simulink model "hoist"  (R2023b)
settings: Solver=FixedStepAuto  StartTime=0.0  StopTime=10.0  FixedStep=0.001  RelTol=1e-3
undefined symbols (not defined in the file): b_hb, b_hEb, b_hwu, bh_eq, i_h, Jh_eq, K_hwu, L_h0, r_hd, T_hb_max, T_hEb_max, Y_t0
settings Model: Creator=Ferran  LastModifiedBy=Ferran
settings DebuggingCC: AlgebraicLoopMsg=none  ArtificialAlgebraicLoopMsg=none
settings ModelReferenceCC: ModelReferenceMinAlgLoopOccurrences=on

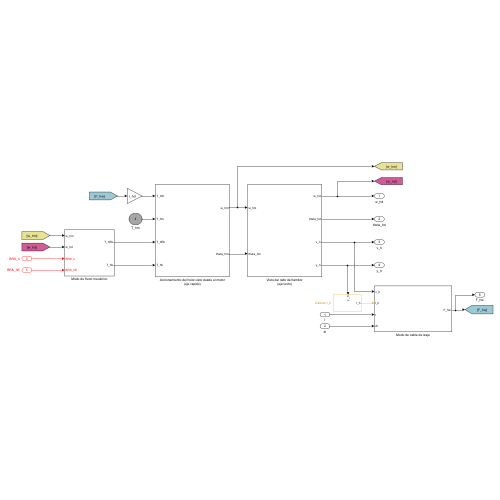
[thumbnail: Simulink's stored preview of the top-level diagram]
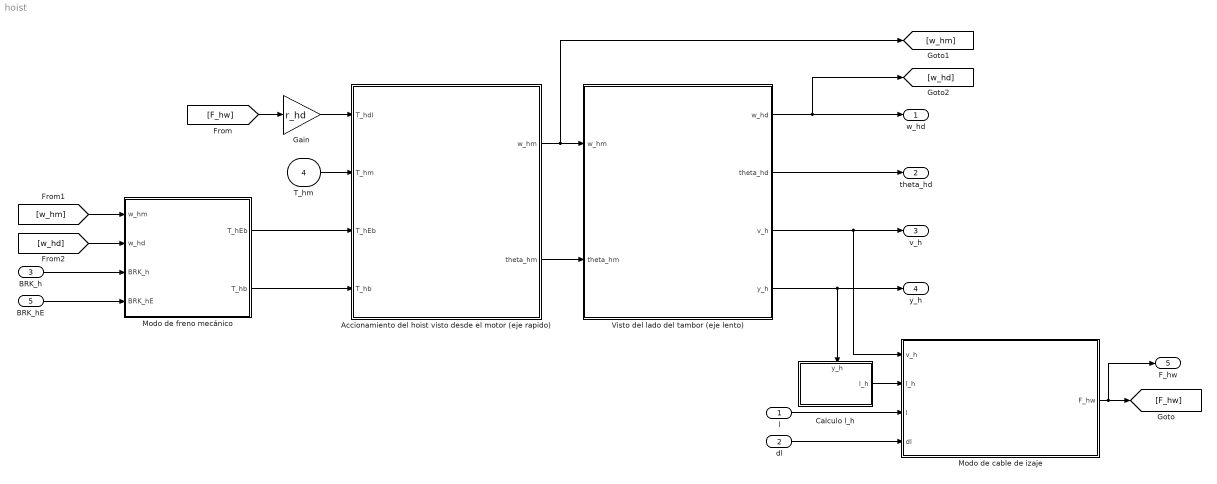
== system hoist ==
  l : Inport
  dl : Inport  Port=2
  BRK_h : Inport  Port=3
  T_hm : Inport  Port=4
  BRK_hE : Inport  Port=5
  Accionamiento del hoist visto desde el motor (eje rapido) : Subsystem
  Calculo l_h : Subsystem
      settings: PortSchema="{\"entries\":[{\"content\":{\"sides\":[{\"content\":{\"connectorIds\":[\"Out1\"]},\"type\":\"ConnectorPlacement.EquallySpacedRectSide\",\"uuid\":\"07ea2d8b-a4bd-4a00-9f3e-d3723522cead\"},{\"content\":{\"side\":\"RIGHT\"},\"type\":\"ConnectorPlacement.EquallySpacedRectSide\",\"uuid\":\"e7371649-c13b-4c3e-a52c-6db8f2f471a9\"},{\"content\":{\"side\":\"TOP\"},\"type\":\"ConnectorPlacement.EquallySpacedRectSide\",\"uuid\":\"bf44ddc9-8ab8-43a2-b974-62ce3b2d20dc\"},{\"content\":{\"connectorIds\":[\"In1\"],\"side\":\"BOTTOM\"},\"type\":\"ConnectorPlacement.EquallySpacedRectSide\",\"uuid\":\"68df679a-1ec0-4ce0-a9ee-39677e661654\"}]},\"type\":\"ConnectorPlacement.EquallySpacedConnector\",\"uuid\":\"345e5710-5df9-4bf4-96c9-62f27951d1e0\"}],\"packageUris\":[\"http://schema.mathworks.com/mf0/Connector/R2020b\"],\"version\":\"1.0\"}"
  Gain : Gain  Gain=r_hd
  Modo de cable de izaje : Subsystem
  Modo de freno mecánico : Subsystem
  Visto del lado del tambor (eje lento) : Subsystem
  w_hd : Outport
  theta_hd : Outport  Port=2
  v_h : Outport  Port=3
  y_h : Outport  Port=4
  F_hw : Outport  Port=5
  wires:
  Accionamiento del hoist visto desde el motor (eje rapido)/2(theta_hm) -> Visto del lado del tambor (eje lento)/2(theta_hm)
  Accionamiento del hoist visto desde el motor (eje rapido)/1(w_hm) -> Visto del lado del tambor (eje lento)/1(w_hm), [w_hm]
  Visto del lado del tambor (eje lento)/4(y_h) -> y_h/1, Calculo l_h/1(y_h)
  l/1 -> Modo de cable de izaje/3(l)
  Calculo l_h/1(l_h) -> Modo de cable de izaje/2(l_h)
  Visto del lado del tambor (eje lento)/3(v_h) -> v_h/1, Modo de cable de izaje/1(v_h)
  Modo de cable de izaje/1(F_hw) -> F_hw/1, [F_hw]
  [F_hw] -> Gain/1
  Gain/1 -> Accionamiento del hoist visto desde el motor (eje rapido)/1(T_hdl)
  dl/1 -> Modo de cable de izaje/4(dl)
  T_hm/1 -> Accionamiento del hoist visto desde el motor (eje rapido)/2(T_hm)
  Visto del lado del tambor (eje lento)/1(w_hd) -> [w_hd], w_hd/1
  Visto del lado del tambor (eje lento)/2(theta_hd) -> theta_hd/1
  BRK_hE/1 -> Modo de freno mecánico/4(BRK_hE)
  [w_hd] -> Modo de freno mecánico/2(w_hd)
  BRK_h/1 -> Modo de freno mecánico/3(BRK_h)
  [w_hm] -> Modo de freno mecánico/1(w_hm)
  Modo de freno mecánico/1(T_hEb) -> Accionamiento del hoist visto desde el motor (eje rapido)/3(T_hEb)
  Modo de freno mecánico/2(T_hb) -> Accionamiento del hoist visto desde el motor (eje rapido)/4(T_hb)

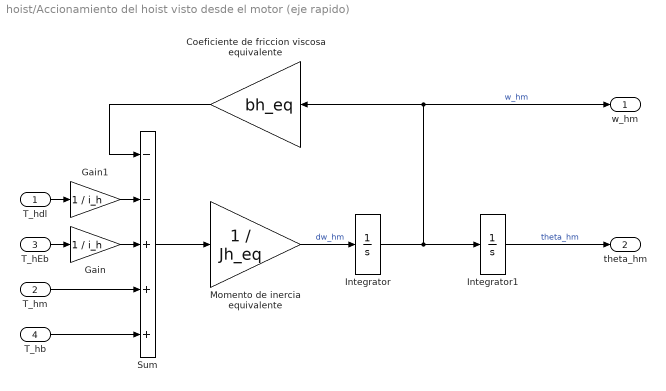
== system hoist/Accionamiento del hoist visto desde el motor (eje rapido) ==
  T_hdl : Inport
  T_hm : Inport  Port=2
  T_hEb : Inport  Port=3
  T_hb : Inport  Port=4
  Coeficiente de friccion viscosa equivalente : Gain  Gain=bh_eq
  Gain : Gain  Gain=1 / i_h
  Gain1 : Gain  Gain=1 / i_h
  Integrator : Integrator
  Integrator1 : Integrator
  Momento de inercia equivalente : Gain  Gain=1 / Jh_eq
  Sum : Sum  Inputs=--+++
  w_hm : Outport
  theta_hm : Outport  Port=2
  wires:
  Integrator1/1 -> theta_hm/1  "theta_hm"
  Coeficiente de friccion viscosa equivalente/1 -> Sum/1
  T_hm/1 -> Sum/4
  Momento de inercia equivalente/1 -> Integrator/1  "dw_hm"
  T_hEb/1 -> Gain/1
  Integrator/1 -> Coeficiente de friccion viscosa equivalente/1, w_hm/1, Integrator1/1  "w_hm"
  T_hb/1 -> Sum/5
  Sum/1 -> Momento de inercia equivalente/1
  T_hdl/1 -> Gain1/1
  Gain/1 -> Sum/3
  Gain1/1 -> Sum/2

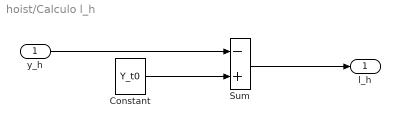
== system hoist/Calculo l_h ==
  y_h : Inport
  Constant : Constant  Value=Y_t0
  Sum : Sum  Inputs=-+
  l_h : Outport
  wires:
  Constant/1 -> Sum/2
  Sum/1 -> l_h/1
  y_h/1 -> Sum/1

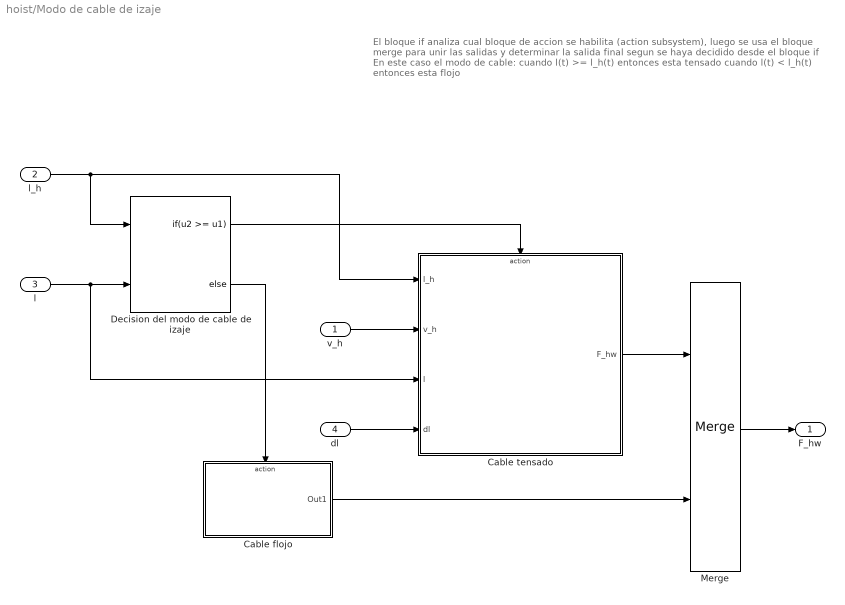
== system hoist/Modo de cable de izaje ==
  note: El bloque if analiza cual bloque de accion se habilita (action subsystem), luego se usa el bloque merge para unir las salidas y determinar la salida final segun se haya decidido desde el bloque if
      |
      | En este caso el modo de cable:
      | cuando l(t) >= l_h(t) entonces esta tensado
      | cuando l(t) < l_h(t) entonces esta flojo
  v_h : Inport
  l_h : Inport  Port=2
  l : Inport  Port=3
  dl : Inport  Port=4
  Cable flojo : Subsystem  TreatAsAtomicUnit=on
  Cable tensado : Subsystem  TreatAsAtomicUnit=on
  Decision del modo de cable de izaje : If  NumInputs=2  IfExpression=u2 >= u1
  Merge : Merge
  F_hw : Outport
  wires:
  Decision del modo de cable de izaje/1 -> Cable tensado/Action
  Decision del modo de cable de izaje/2 -> Cable flojo/Action
  l/1 -> Decision del modo de cable de izaje/2, Cable tensado/3(l)
  Cable flojo/1(Out1) -> Merge/2
  dl/1 -> Cable tensado/4(dl)
  l_h/1 -> Decision del modo de cable de izaje/1, Cable tensado/1(l_h)
  Cable tensado/1(F_hw) -> Merge/1
  v_h/1 -> Cable tensado/2(v_h)
  Merge/1 -> F_hw/1

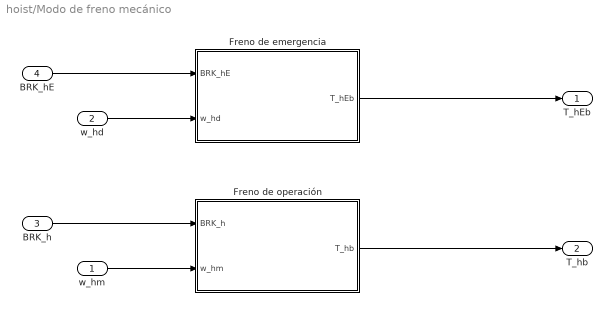
== system hoist/Modo de freno mecánico ==
  w_hm : Inport
  w_hd : Inport  Port=2
  BRK_h : Inport  Port=3
  BRK_hE : Inport  Port=4
  Freno de emergencia : Subsystem
  Freno de operación : Subsystem
  T_hEb : Outport
  T_hb : Outport  Port=2
  wires:
  w_hm/1 -> Freno de operación/2(w_hm)
  BRK_hE/1 -> Freno de emergencia/1(BRK_hE)
  Freno de operación/1(T_hb) -> T_hb/1
  Freno de emergencia/1(T_hEb) -> T_hEb/1
  w_hd/1 -> Freno de emergencia/2(w_hd)
  BRK_h/1 -> Freno de operación/1(BRK_h)

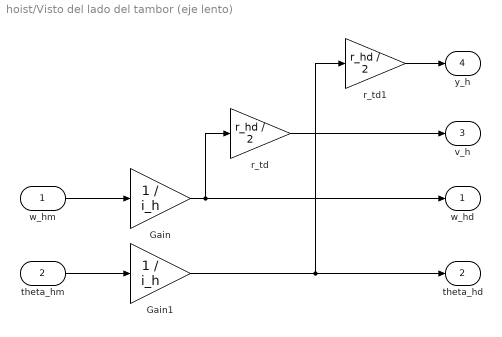
== system hoist/Visto del lado del tambor (eje lento) ==
  w_hm : Inport
  theta_hm : Inport  Port=2
  Gain : Gain  Gain=1 / i_h
  Gain1 : Gain  Gain=1 / i_h
  r_td : Gain  Gain=r_hd / 2
  r_td1 : Gain  Gain=r_hd / 2
  w_hd : Outport
  theta_hd : Outport  Port=2
  v_h : Outport  Port=3
  y_h : Outport  Port=4
  wires:
  Gain1/1 -> r_td1/1, theta_hd/1
  Gain/1 -> w_hd/1, r_td/1
  w_hm/1 -> Gain/1
  theta_hm/1 -> Gain1/1
  r_td/1 -> v_h/1
  r_td1/1 -> y_h/1

== system hoist/Modo de cable de izaje/Cable flojo ==
  Action Port : ActionPort  ActionPortLabel=else
  Zero : Constant  Value=0  OutDataTypeStr=Inherit: Inherit via back propagation
  Out1 : Outport
  wires:
  Zero/1 -> Out1/1

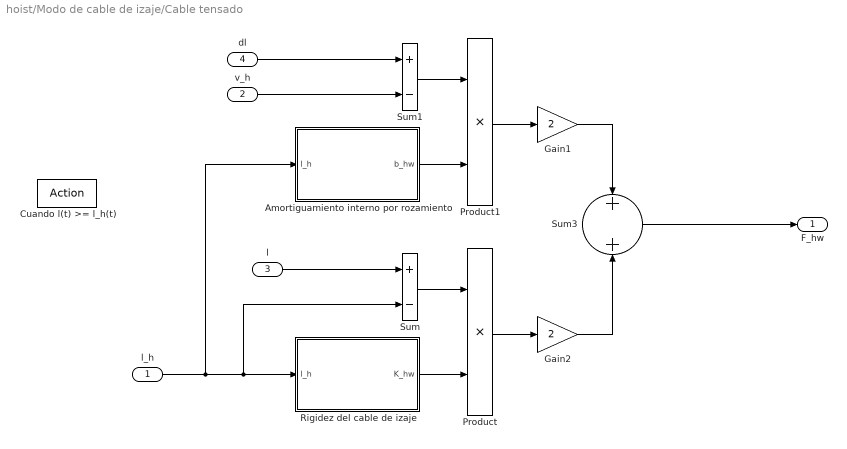
== system hoist/Modo de cable de izaje/Cable tensado ==
  l_h : Inport
  v_h : Inport  Port=2
  l : Inport  Port=3
  dl : Inport  Port=4
  Cuando l(t) >= l_h(t) : ActionPort  ActionPortLabel=if(u2 >= u1)
  Amortiguamiento interno por rozamiento : Subsystem
  Gain1 : Gain  Gain=2
  Gain2 : Gain  Gain=2
  Product : Product
  Product1 : Product
  Rigidez del cable de izaje : Subsystem
  Sum : Sum  Inputs=+-
  Sum1 : Sum  Inputs=+-
  Sum3 : Sum
  F_hw : Outport
  wires:
  l/1 -> Sum/1
  l_h/1 -> Amortiguamiento interno por rozamiento/1(l_h), Rigidez del cable de izaje/1(l_h), Sum/2
  Sum3/1 -> F_hw/1
  Gain1/1 -> Sum3/1
  Gain2/1 -> Sum3/2
  Rigidez del cable de izaje/1(K_hw) -> Product/2
  Amortiguamiento interno por rozamiento/1(b_hw) -> Product1/2
  Sum1/1 -> Product1/1
  Sum/1 -> Product/1
  v_h/1 -> Sum1/2
  Product1/1 -> Gain1/1
  Product/1 -> Gain2/1
  dl/1 -> Sum1/1

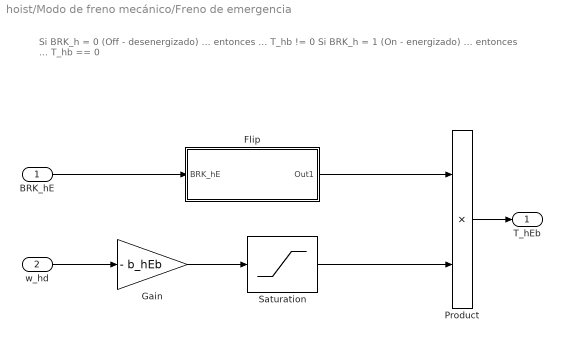
== system hoist/Modo de freno mecánico/Freno de emergencia ==
  note: Si BRK_h = 0 (Off - desenergizado) ... entonces ... T_hb != 0
      | Si BRK_h = 1 (On - energizado) ... entonces ... T_hb == 0
  BRK_hE : Inport
  w_hd : Inport  Port=2
  Flip : Subsystem
  Gain : Gain  Gain=- b_hEb
  Product : Product
  Saturation : Saturate  UpperLimit=T_hEb_max  LowerLimit=-T_hEb_max
  T_hEb : Outport
  wires:
  w_hd/1 -> Gain/1
  BRK_hE/1 -> Flip/1(BRK_hE)
  Product/1 -> T_hEb/1
  Gain/1 -> Saturation/1
  Flip/1(Out1) -> Product/1
  Saturation/1 -> Product/2

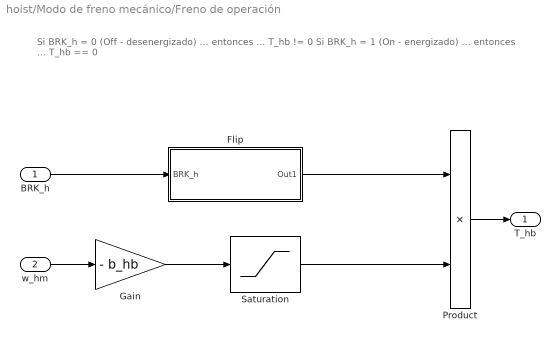
== system hoist/Modo de freno mecánico/Freno de operación ==
  note: Si BRK_h = 0 (Off - desenergizado) ... entonces ... T_hb != 0
      | Si BRK_h = 1 (On - energizado) ... entonces ... T_hb == 0
  BRK_h : Inport
  w_hm : Inport  Port=2
  Flip : Subsystem
  Gain : Gain  Gain=- b_hb
  Product : Product
  Saturation : Saturate  UpperLimit=T_hb_max  LowerLimit=-T_hb_max
  T_hb : Outport
  wires:
  w_hm/1 -> Gain/1
  BRK_h/1 -> Flip/1(BRK_h)
  Product/1 -> T_hb/1
  Flip/1(Out1) -> Product/1
  Saturation/1 -> Product/2
  Gain/1 -> Saturation/1

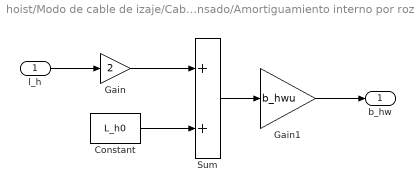
== system hoist/Modo de cable de izaje/Cable tensado/Amortiguamiento interno por rozamiento ==
  l_h : Inport
  Constant : Constant  Value=L_h0
  Gain : Gain  Gain=2
  Gain1 : Gain  Gain=b_hwu
  Sum : Sum
  b_hw : Outport
  wires:
  Sum/1 -> Gain1/1
  Gain/1 -> Sum/1
  Gain1/1 -> b_hw/1
  Constant/1 -> Sum/2
  l_h/1 -> Gain/1

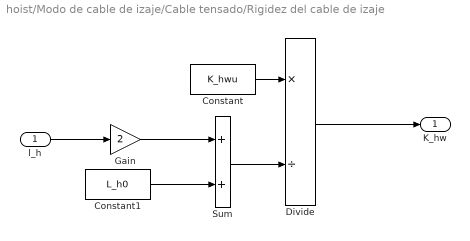
== system hoist/Modo de cable de izaje/Cable tensado/Rigidez del cable de izaje ==
  l_h : Inport
  Constant : Constant  Value=K_hwu
  Constant1 : Constant  Value=L_h0
  Divide : Product  Inputs=*/
  Gain : Gain  Gain=2
  Sum : Sum
  K_hw : Outport
  wires:
  Constant1/1 -> Sum/2
  Sum/1 -> Divide/2
  Gain/1 -> Sum/1
  Constant/1 -> Divide/1
  Divide/1 -> K_hw/1
  l_h/1 -> Gain/1

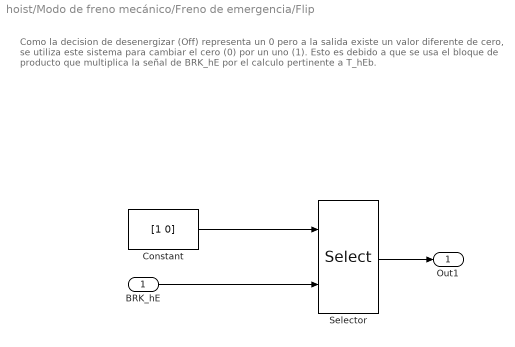
== system hoist/Modo de freno mecánico/Freno de emergencia/Flip ==
  note: Como la decision de desenergizar (Off) representa un 0 pero a la salida existe un valor diferente de cero, se utiliza este sistema para cambiar el cero (0) por un uno (1).
      |
      | Esto es debido a que se usa el bloque de producto que multiplica la señal de BRK_hE por el calculo pertinente a T_hEb.
  BRK_hE : Inport
  Constant : Constant  Value=[1 0]
  Selector : Selector  IndexMode=Zero-based  InputPortWidth=2  IndexOptions=Starting index (port)  Indices=[1 3]  OutputSizes=1
  Out1 : Outport
  wires:
  BRK_hE/1 -> Selector/2
  Constant/1 -> Selector/1
  Selector/1 -> Out1/1

== system hoist/Modo de freno mecánico/Freno de operación/Flip ==
  note: Como la decision de desenergizar (Off) representa un 0 pero a la salida existe un valor diferente de cero, se utiliza este sistema para cambiar el cero (0) por un uno (1).
      |
      | Esto es debido a que se usa el bloque de producto que multiplica la señal de BRK_h por el calculo pertinente a T_hb.
  BRK_h : Inport
  Constant : Constant  Value=[1 0]
  Selector : Selector  IndexMode=Zero-based  InputPortWidth=2  IndexOptions=Starting index (port)  Indices=[1 3]  OutputSizes=1
  Out1 : Outport
  wires:
  BRK_h/1 -> Selector/2
  Constant/1 -> Selector/1
  Selector/1 -> Out1/1
